simulink model "35 Bus Network Electricity Transmission Model"  (R2023b)
settings: Solver=VariableStepAuto  StartTime=0.0  StopTime=1  RelTol=1e-3
model workspace (MAT data in the model file):
  T_set = 0.0001
  Tp = 5e-05
undefined symbols (not defined in the file): D1, D11, Delta, DiscIntNeverNeededParam
libraries: spsSeriesRLCBranchLib x57, spsLoadFlowBusLib x35, spsThreePhaseSeriesRLCLoadLib x28, spsThreePhaseTransformerTwoWindingsLib x22, spsDistributedParametersLineLib x22, spsGenericPowerSystemStabilizerLib x20, spsThreePhaseVIMeasurementLib x14, spsSynchronousMachinepuStandardLib x10, spsExcitationSystemLib x10, spsHydraulicTurbineandGovernorLib x10, spsFourierLib x8, spsMeanLib x8
(part 1 of 8)
settings Model: Creator=3.22  LastModifiedBy=3.22

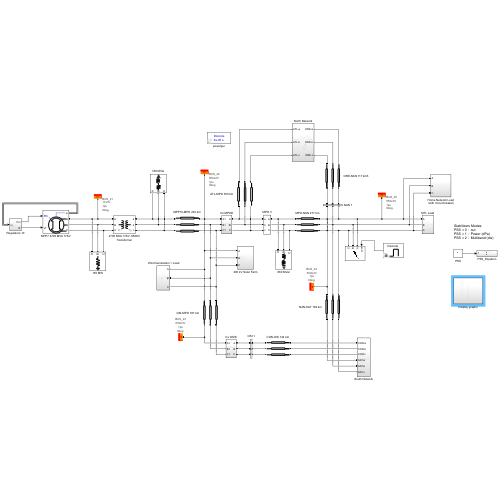
[thumbnail: Simulink's stored preview of the top-level diagram]
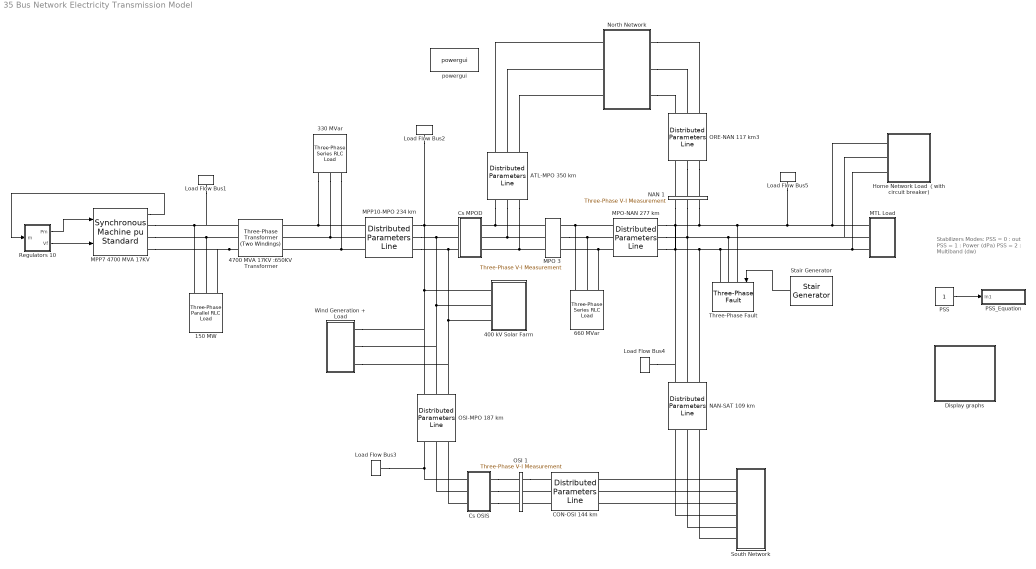
== system 35 Bus Network Electricity Transmission Model ==
  note: Stabilizers Modes:
      | PSS = 0 :  out
      | PSS = 1 :  Power (dPa)
      | PSS = 2 :  Multiband (dw)
  " Wind Generation + Load" : Subsystem
  150 MW : spsThreePhaseParallelRLCLoadLib/Three-Phase Parallel RLC Load  LConnTagsString=A|B|C  Configuration=Y (grounded)  NominalVoltage=17000  Vabc=[1e3 1e3 1e3]  Vabcp=[1e3 1e3 1e3]  NominalFrequency=60  UnbalancedPower=off  ActivePower=150e6  InductivePower=0  CapacitivePower=0  Pabc=[10e3 9e3 11e3]  QLabc=[100 90 110]  QCabc=[100 90 110]  Pabcp=[10e3 9e3 11e3]  QLabcp=[100 90 110]  QCabcp=[100 90 110]  Measurements=None  LoadType=constant Z
  330 MVar : spsThreePhaseSeriesRLCLoadLib/Three-Phase Series RLC Load  LConnTagsString=A|B|C  Configuration=Y (grounded)  NominalVoltage=650e3  Vabc=[1e3 1e3 1e3]  Vabcp=[1e3 1e3 1e3]  NominalFrequency=60  UnbalancedPower=off  ActivePower=1100e3  InductivePower=330e6  CapacitivePower=0  Pabc=[10e3 9e3 11e3]  QLabc=[100 90 110]  QCabc=[100 90 110]  Pabcp=[10e3 9e3 11e3]  QLabcp=[100 90 110]  QCabcp=[100 90 110]  Measurements=None  LoadType=constant Z
  400 kV Solar Farm : Subsystem
  "4700 MVA 17KV :650KV Transformer " : spsThreePhaseTransformerTwoWindingsLib/Three-Phase Transformer (Two Windings)  Winding1Connection=Delta (D1)  Winding2Connection=Yg  CoreType=Three single-phase transformers  SetSaturation=off  Hysteresis=off  DataFile='hysteresis'  SetInitialFlux=off  Measurements=None  UNITS=pu  NominalPower=[ 4700e6 , 60 ]  Winding1=[ 17e3 , 0.002 , 0.08 ]  Winding2=[ 650e3 , 0.002 , 0.08 ]  Rm=500  Lm=500  L0=0.5  Saturation=[ 0,0 ; 0.0024,1.2 ; 1.0,1.52 ]  InitialFluxes=[ 0.8 , -0.8 , 0.7 ]  BreakLoop=off  DiscreteSolver=Trapezoidal iterative  DataType=off  TransfoNumber=1
  660 MVar : spsThreePhaseSeriesRLCLoadLib/Three-Phase Series RLC Load  LConnTagsString=A|B|C  Configuration=Y (grounded)  NominalVoltage=650e3  Vabc=[1e3 1e3 1e3]  Vabcp=[1e3 1e3 1e3]  NominalFrequency=60  UnbalancedPower=off  ActivePower=2200e3  InductivePower=660e6  CapacitivePower=0  Pabc=[10e3 9e3 11e3]  QLabc=[100 90 110]  QCabc=[100 90 110]  Pabcp=[10e3 9e3 11e3]  QLabcp=[100 90 110]  QCabcp=[100 90 110]  Measurements=None  LoadType=constant Z
  ATL-MPO 350 km : spsDistributedParametersLineLib/Distributed Parameters Line  Phases=3  Length=350  Frequency=60  Resistance=[0.01273 0.3864]/6  Inductance="[0.9337e-3  4.1264e-3]/6"  Capacitance=[12.74e-9 7.751e-9]*6  x1=[-0.00198 -4.66537973862611e-08 -283995.035900817 -140929.158887352;-0.00192 -4.56218918231529e-08 -280734.893310355 -147316.404665037;-0.00186 -4.45666452571923e-08 -277331.121561091 -153628.280648;-0.0018 -4.34885975720212e-08 -273785.462085546 -159861.557563859;-0.00174 -4.23883003167554e-08 -270099.728908624 -166013.046352967;-0.00168 -4.12663164238018e-08 -266275.807719524 -172079.599799993;-0.00162 -4.0123219920852e-08 -262315.654906983 -178058.114144095;-0.00156 -3.89595956371987e-08 -258221.296558356 -183945.530666865;-0.0015 -3.77760389045269e-08 -253994.827423029 -189738.837257224;-0.00144 -3.65731552523307e-08 -249638.409840707 -195435.069952471;-0.00138 -3.53515600981131e-08 -245154.272635124 -201031.314454706;-0.00132 -3.41118784325276e-08 -240544.70997373 -206524.707621834;-0.00126 -3.2854744499621e-08 -235812.080193958 -211912.438932405;-0.0012 -3.15808014723424e-08 -230958.804596653 -217191.751923527;-0.00114 -3.02907011234846e-08 -225987.366207288 -222359.945601122;-0.00108 -2.89851034922241e-08 -220900.308505605 -227414.375821808;-0.00102 -2.76646765464339e-08 -215700.234124322 -232352.45664569;-0.00096 -2.63300958409381e-08 -210389.803517579 -237171.661659371;-0.0009 -2.49820441718858e-08 -204971.7335998 -241869.52526852;-0.00084 -2.36212112274201e-08 -199448.796355669 -246443.643959306;-0.00078 -2.22482932348207e-08 -193823.817421933 -250891.677528087;-0.00072 -2.08639926043011e-08 -188099.674641751 -255211.3502787;-0.00066 -1.94690175696429e-08 -182279.29659234 -259400.452186747;-0.0006 -1.806408182585e-08 -176365.661086658 -263456.840030286;-0.00054 -1.66499041640091e-08 -170361.793649902 -267378.438486342;-0.00048 -1.52272081035431e-08 -164270.76597159 -271163.241192684;-0.00042 -1.37967215220448e-08 -158095.694334033 -274809.31177431;-0.00036 -1.23591762828818e-08 -151839.738017982 -278314.784834141;-0.0003 -1.09153078607611e-08 -145506.097686284 -281677.866907385;-0.00024 -9.46585496544719e-09 -139098.013746368 -284896.83737911;-0.00018 -8.01155916382403e-09 -132618.764692382 -287970.049364544;-0.00012 -6.55316450049607e-09 -126071.665427867 -290895.930551648;-6e-05 -5.0914171171211e-09 -119460.065569783 -293672.984005544]  x2=[-0.00198 -4.73470407763487e-08 -244678.153400783 -153858.077281588;-0.00192 -4.70683207225062e-08 -241135.650149882 -159352.765994398;-0.00186 -4.67655196460595e-08 -237469.77744469 -164765.926887624;-0.0018 -4.64387924656344e-08 -233682.41081342 -170094.790488131;-0.00174 -4.60883063408937e-08 -229775.487942824 -175336.630450834;-0.00168 -4.5714240587015e-08 -225751.007686833 -180488.764953549;-0.00162 -4.53167865829499e-08 -221611.02904391 -185548.558069066;-0.00156 -4.48961476735111e-08 -217357.670103628 -190513.421113731;-0.0015 -4.44525390653371e-08 -212993.106963013 -195380.813971871;-0.00144 -4.39861877167887e-08 -208519.572613215 -200148.24639536;-0.00138 -4.34973322218332e-08 -203939.35579707 -204813.27927768;-0.00132 -4.29862226879746e-08 -199254.799838133 -209373.525901807;-0.00126 -4.24531206082949e-08 -194468.301441793 -213826.653161304;-0.0012 -4.18982987276684e-08 -189582.309469075 -218170.382753982;-0.00114 -4.13220409032214e-08 -184599.323683754 -222402.492347517;-0.00108 -4.07246419591047e-08 -179521.893473433 -226520.816716443;-0.00102 -4.01064075356569e-08 -174352.616545228 -230523.248849912;-0.00096 -3.94676539330326e-08 -169094.137596732 -234407.74102969;-0.0009 -3.88087079493778e-08 -163749.146962942 -238172.305877801;-0.00084 -3.81299067136336e-08 -158320.379239828 -241815.017373306;-0.00078 -3.74315975130551e-08 -152810.611885272 -245334.011837695;-0.00072 -3.67141376155325e-08 -147222.66379806 -248727.488888376;-0.00066 -3.59778940868065e-08 -141559.393875686 -251993.712359787;-0.0006 -3.52232436026707e-08 -135823.699551689 -255131.011191646;-0.00054 -3.4450572256257e-08 -130018.515313268 -258137.7802839;-0.00048 -3.36602753605036e-08 -124146.811199946 -261012.481317923;-0.00042 -3.28527572459055e-08 -118211.591284045 -263753.643543548;-0.00036 -3.20284310536511e-08 -112215.892133745 -266359.864531529;-0.0003 -3.11877185242524e-08 -106162.781259517 -268829.810891052;-0.00024 -3.03310497817739e-08 -100055.355544735 -271162.218951918;-0.00018 -2.94588631137736e-08 -93896.739661245 -273355.895411067;-0.00012 -2.85716047470672e-08 -87690.0844707324 -275409.717943088;-6e-05 -2.76697286194296e-08 -81438.5654126781 -277322.635774423]  x3=[-0.00198 -1.15739742869573e-10 -7510.86676188477 -3625.13536494991;-0.00192 -1.13432270648557e-10 -7426.95305478795 -3794.08593924927;-0.00186 -1.11066764381889e-10 -7339.23958127399 -3961.09538907547;-0.0018 -1.08644434306286e-10 -7247.7712171767 -4126.07826930798;-0.00174 -1.06166519730574e-10 -7152.59475940128 -4288.95017165676;-0.00168 -1.03634288401635e-10 -7053.7589019822 -4449.62776784703;-0.00162 -1.01049035855809e-10 -6951.31421117039 -4608.02885225161;-0.00156 -9.84120847560678e-11 -6845.31309956262 -4764.07238394879;-0.0015 -9.57247842153189e-11 -6735.80979928628 -4917.6785281844;-0.00144 -9.29885091061748e-11 -6622.86033425316 -5068.76869721674;-0.00138 -9.02046593575419e-11 -6506.52249149665 -5217.26559052351;-0.00132 -8.73746592383912e-11 -6386.85579160679 -5363.09323435019;-0.00126 -8.4499956629076e-11 -6263.9214582784 -5506.1770205796;-0.0012 -8.15820222805698e-11 -6137.78238698801 -5646.44374490283;-0.00114 -7.86223490620024e-11 -6008.50311281525 -5783.82164427189;-0.00108 -7.56224511968808e-11 -5876.1497774256 -5918.240433615;-0.00102 -7.25838634883847e-11 -5740.79009523106 -6049.63134179576;-0.00096 -6.95081405341324e-11 -5602.49331874619 -6177.92714679772;-0.0009 -6.63968559308201e-11 -5461.33020315728 -6303.06221011642;-0.00084 -6.32516014691407e-11 -5317.37297012266 -6424.97251034122;-0.00078 -6.00739863193944e-11 -5170.69527082276 -6543.59567590988;-0.00072 -5.68656362082076e-11 -5021.37214827885 -6658.87101701901;-0.00066 -5.36281925867804e-11 -4869.47999895959 -6770.73955667404;-0.0006 -5.03633117910908e-11 -4715.09653369522 -6879.14406086299;-0.00054 -4.70726641944819e-11 -4558.30073791924 -6984.02906783844;-0.00048 -4.37579333530683e-11 -4399.17283125803 -7085.34091649276;-0.00042 -4.04208151443976e-11 -4237.79422648898 -7183.02777381216;-0.00036 -3.70630168998082e-11 -4074.24748788822 -7277.03966139538;-0.0003 -3.3686256530927e-11 -3908.61628898922 -7367.3284810236;-0.00024 -3.02922616507542e-11 -3740.98536977385 -7453.84803926836;-0.00018 -2.68827686897843e-11 -3571.44049331784 -7536.55407112494;-0.00012 -2.34595220076162e-11 -3400.06840191282 -7615.40426265923;-6e-05 -2.00242730005068e-11 -3226.95677268734 -7690.35827265625]  x4=[-0.00198 -7.16737734589059e-10 -5560.43523467954 -135.899816413835;-0.00192 -7.1591261080325e-10 -5555.93855175485 -261.62884284291;-0.00186 -7.1472121289721e-10 -5548.59934800515 -387.224015121641;-0.0018 -7.13164150412122e-10 -5538.42137830268 -512.621076439158;-0.00174 -7.11242219969926e-10 -5525.40984988481 -637.755871341821;-0.00168 -7.08956404865747e-10 -5509.5714196899 -762.564378556332;-0.00162 -7.06307874564831e-10 -5490.91419095151 -886.982743744204;-0.00156 -7.03297984104218e-10 -5469.44770905259 -1010.94731217082;-0.0015 -6.99928273399485e-10 -5445.18295664195 -1134.39466127237;-0.00144 -6.96200466456894e-10 -5418.13234801529 -1257.26163310401;-0.00138 -6.92116470491358e-10 -5388.3097227638 -1379.48536665263;-0.00132 -6.87678374950676e-10 -5355.73033869363 -1501.00332999771;-0.00126 -6.82888450446534e-10 -5320.41086401966 -1621.75335230382;-0.0012 -6.77749147592816e-10 -5282.36936883778 -1741.67365562832;-0.00114 -6.72263095751826e-10 -5241.62531587983 -1860.70288652818;-0.00108 -6.66433101689054e-10 -5198.19955055618 -1978.78014744946;-0.00102 -6.60262148137191e-10 -5152.11429029078 -2095.84502788364;-0.00096 -6.53753392270099e-10 -5103.39311315434 -2211.8376352748;-0.0009 -6.46910164087548e-10 -5052.06094580135 -2326.69862566169;-0.00084 -6.39735964711525e-10 -4998.14405071713 -2440.36923403925;-0.00078 -6.32234464594993e-10 -4941.67001278149 -2552.79130442383;-0.00072 -6.24409501644025e-10 -4882.66772515574 -2663.90731960691;-0.00066 -6.16265079254255e-10 -4821.16737450048 -2773.66043058193;-0.0006 -6.07805364262669e-10 -4757.20042553149 -2881.99448562931;-0.00054 -5.99034684815774e-10 -4690.79960492184 -2988.85405904471;-0.00048 -5.89957528155239e-10 -4621.9988845583 -3094.18447949583;-0.00042 -5.80578538322139e-10 -4550.83346416071 -3197.93185799329;-0.00036 -5.70902513780975e-10 -4477.33975327311 -3300.0431154612;-0.0003 -5.60934404964694e-10 -4401.55535263602 -3400.46600989346;-0.00024 -5.50679311741958e-10 -4323.51903494912 -3499.14916308168;-0.00018 -5.40142480807951e-10 -4243.2707250345 -3596.04208690122;-0.00012 -5.29329303000077e-10 -4160.85147941032 -3691.09520914188;-6e-05 -5.18245310539908e-10 -4076.30346528558 -3784.25989886994]  x5=0.0019793954844851  V1=[4.219e-16 0.0001256 0.0001256;377 377 377;2.896 1.02 -0.5506]  V2=[3.447e-16 8.016e-05 8.016e-05;377 377 377;2.788 1.015 -0.5555]  I1=[4.128e-19 5.188e-07 5.188e-07;377 377 377;2.697 1.572 0.0007381]  I2=[5.884e-19 5.436e-07 5.436e-07;377 377 377;2.289 0.05248 -1.518]  nHarmo=1  Measurements=None  Decoupling=off  VsMag0=0  VrMag0=0  VsAngle0=0  VrAngle0=0  IsMag0=0  IrMag0=0  IsAngle0=0  IrAngle0=0
      settings: LibrarySourceBlock=sps_lib/Power Grid Elements/Distributed Parameters Line
  CON-OSI 144 km : spsDistributedParametersLineLib/Distributed Parameters Line  Phases=3  Length=144  Frequency=60  Resistance=[0.01273 0.3864]/6  Inductance="[0.9337e-3  4.1264e-3]/6"  Capacitance=[12.74e-9 7.751e-9]*6  x1=[-0.00084 1.58878300947761e-08 0 0;-0.00078 1.81135659339013e-08 0 0;-0.00072 2.03300345379945e-08 0 0;-0.00066 2.25361019207623e-08 0 0;-0.0006 2.4730639417368e-08 0 0;-0.00054 2.69125242618782e-08 -153418.27699203 -260460.282018713;-0.00048 2.90806401616898e-08 -147488.056603015 -263863.63509505;-0.00042 3.12338778686461e-08 -141482.378598976 -267131.990660033;-0.00036 3.33711357465492e-08 -135404.315595752 -270263.676562563;-0.0003 3.54913203347766e-08 -129256.977242685 -273257.090574265;-0.00024 3.75933469077166e-08 -123043.508631666 -276110.701209219;-0.00018 3.96761400297334e-08 -116767.088688049 -278823.048507495;-0.00012 4.17386341053802e-08 -110430.928544252 -281392.744782097;-6e-05 4.37797739245774e-08 -104038.269896882 -283818.475328928]  x2=[-0.00084 2.59938982630843e-08 0 0;-0.00078 2.7994091738396e-08 0 0;-0.00072 2.9979962919103e-08 0 0;-0.00066 3.19504957968145e-08 0 0;-0.0006 3.39046822104992e-08 0 0;-0.00054 3.58415223622784e-08 -143552.051614192 -254203.94929145;-0.00048 3.77600253289419e-08 -137765.858511586 -257385.752758705;-0.00042 3.9659209568922e-08 -131909.181850144 -260435.872918908;-0.00036 4.15381034244688e-08 -125985.018013867 -263352.749274224;-0.0003 4.33957456187677e-08 -119996.397914438 -266134.889496811;-0.00024 4.52311857477469e-08 -113946.385440558 -268780.870192325;-0.00018 4.70434847663213e-08 -107838.075890399 -271289.337628149;-0.00012 4.88317154688256e-08 -101674.594387996 -273659.008425992;-6e-05 5.05949629633897e-08 -95459.0942843738 -275888.670218487]  x3=[-0.00084 3.07553029750544e-10 0 0;-0.00078 3.29548959067833e-10 0 0;-0.00072 3.51376285048298e-10 0 0;-0.00066 3.73023840428645e-10 0 0;-0.0006 3.94480549919541e-10 0 0;-0.00054 4.15735435871936e-10 -3139.71318404474 -6567.77181842436;-0.00048 4.3677762389343e-10 -2990.36305476603 -6637.10518863291;-0.00042 4.57596348411819e-10 -2839.48300049295 -6703.04289318734;-0.00036 4.78180958182951e-10 -2687.1502142492 -6765.55119713963;-0.0003 4.98520921740109e-10 -2533.44263230302 -6824.59812008645;-0.00024 5.18605832782097e-10 -2378.43889429351 -6880.15345253095;-0.00018 5.384254154973e-10 -2222.21830299718 -6932.18877133853;-0.00012 5.57969529820977e-10 -2064.86078375517 -6980.67745427856;-6e-05 5.77228176623106e-10 -1906.44684358194 -7025.5946936449]  x4=[-0.00084 -2.09296979855395e-10 0 0;-0.00078 -1.97214230323626e-10 0 0;-0.00072 -1.85030582347523e-10 0 0;-0.00066 -1.72752269306518e-10 0 0;-0.0006 -1.60385573012442e-10 0 0;-0.00054 -1.47936820495628e-10 -4476.02404663198 -4165.00505473071;-0.00048 -1.3541238076789e-10 -4380.67668178872 -4265.17699903546;-0.00042 -1.22818661564018e-10 -4283.08808180945 -4363.1667999761;-0.00036 -1.10162106063462e-10 -4183.30817482517 -4458.92432415982;-0.0003 -9.74491895938823e-11 -4081.38801008 -4552.40058026784;-0.00024 -8.46864163182524e-11 -3977.37973181349 -4643.54774412032;-0.00018 -7.1880315907209e-11 -3871.33655258266 -4732.319183144;-0.00012 -5.9037440198352e-11 -3763.31272603746 -4818.66948023038;-6e-05 -4.6164359844203e-11 -3653.36351916359 -4902.55445697191]  x5=0.000814379856473869  V1=[3.066e-13 0.3294 0.3294;377 377 377;-0.5534 -1.851 2.861]  V2=[2.167e-13 0.2213 0.2213;377 377 377;-0.5727 -1.852 2.86]  I1=[4.19e-16 0.002316 0.002316;377 377 377;0.2564 -0.79 -2.361]  I2=[5.677e-16 0.002387 0.002387;377 377 377;-1.374 -3.038 1.674]  nHarmo=1  Measurements=None  Decoupling=off  VsMag0=0  VrMag0=0  VsAngle0=0  VrAngle0=0  IsMag0=0  IrMag0=0  IsAngle0=0  IrAngle0=0
      settings: LibrarySourceBlock=sps_lib/Power Grid Elements/Distributed Parameters Line
  Cs MPOD : Subsystem
  Cs OSIS : Subsystem
  Display graphs : Subsystem
  Home Network Load （with circuit breaker) : Subsystem
  Load Flow Bus1 : spsLoadFlowBusLib/Load Flow Bus  LConnTagsString=a  Phases=single  Connectors=on one side  ID=BUS_21  Vbase=17e3  Vref=1  Vangle=0  VLF=1  VLFb=1  VLFc=1  angleLF=0  angleLFb=0  angleLFc=0
  Load Flow Bus2 : spsLoadFlowBusLib/Load Flow Bus  LConnTagsString=a  Phases=single  Connectors=on one side  ID=BUS_22  Vbase=650e3  Vref=1  Vangle=0  VLF=1  VLFb=1  VLFc=1  angleLF=0  angleLFb=0  angleLFc=0
  Load Flow Bus3 : spsLoadFlowBusLib/Load Flow Bus  LConnTagsString=a  Phases=single  Connectors=on one side  ID=BUS_23  Vbase=650e3  Vref=1  Vangle=0  VLF=1  VLFb=1  VLFc=1  angleLF=0  angleLFb=0  angleLFc=0
  Load Flow Bus4 : spsLoadFlowBusLib/Load Flow Bus  LConnTagsString=a  Phases=single  Connectors=on one side  ID=BUS_24  Vbase=650e3  Vref=1  Vangle=0  VLF=1  VLFb=1  VLFc=1  angleLF=0  angleLFb=0  angleLFc=0
  Load Flow Bus5 : spsLoadFlowBusLib/Load Flow Bus  LConnTagsString=a  Phases=single  Connectors=on one side  ID=BUS_25  Vbase=650e3  Vref=1  Vangle=0  VLF=1  VLFb=1  VLFc=1  angleLF=0  angleLFb=0  angleLFc=0
  MPO 3 : spsThreePhaseVIMeasurementLib/Three-Phase V-I Measurement  VoltageMeasurement=no  SetLabelV=off  LabelV=Vabc_MPO3  Vpu=off  VpuLL=off  CurrentMeasurement=no  SetLabelI=off  LabelI=Iabc  Ipu=off  Pbase=100e6  Vbase=500e3  OutputType=Complex  PhasorSimulation=off  PSBequivalent=0
  MPO-NAN 277 km : spsDistributedParametersLineLib/Distributed Parameters Line  Phases=3  Length=277  Frequency=60  Resistance=[0.01273 0.3864]/6  Inductance="[0.9337e-3  4.1264e-3]/6"  Capacitance=[12.74e-9 7.751e-9]*6  x1=[-0.00162 -4.0123219920852e-08 -262315.654906984 -178058.114144095;-0.00156 -3.89595956371987e-08 -258221.296558356 -183945.530666865;-0.0015 -3.77760389045269e-08 -253994.827423029 -189738.837257224;-0.00144 -3.65731552523307e-08 -249638.409840707 -195435.069952471;-0.00138 -3.53515600981131e-08 -245154.272635124 -201031.314454706;-0.00132 -3.41118784325276e-08 -240544.70997373 -206524.707621834;-0.00126 -3.2854744499621e-08 -235812.080193958 -211912.438932405;-0.0012 -3.15808014723424e-08 -230958.804596653 -217191.751923527;-0.00114 -3.02907011234846e-08 -225987.366207288 -222359.945601122;-0.00108 -2.89851034922241e-08 -220900.308505605 -227414.375821808;-0.00102 -2.76646765464339e-08 -215700.234124322 -232352.45664569;-0.00096 -2.63300958409381e-08 -210389.803517579 -237171.661659371;-0.0009 -2.49820441718858e-08 -204971.7335998 -241869.52526852;-0.00084 -2.36212112274201e-08 -199448.796355669 -246443.643959306;-0.00078 -2.22482932348207e-08 -193823.817421933 -250891.677528087;-0.00072 -2.08639926043011e-08 -188099.674641751 -255211.3502787;-0.00066 -1.94690175696429e-08 -182279.29659234 -259400.452186747;-0.0006 -1.806408182585e-08 -176365.661086658 -263456.840030286;-0.00054 -1.66499041640091e-08 -170361.793649902 -267378.438486342;-0.00048 -1.52272081035431e-08 -164270.76597159 -271163.241192684;-0.00042 -1.37967215220448e-08 -158095.694334033 -274809.31177431;-0.00036 -1.23591762828818e-08 -151839.738017982 -278314.784834141;-0.0003 -1.09153078607611e-08 -145506.097686284 -281677.866907385;-0.00024 -9.46585496544719e-09 -139098.013746368 -284896.83737911;-0.00018 -8.01155916382403e-09 -132618.764692382 -287970.049364544;-0.00012 -6.55316450049607e-09 -126071.665427867 -290895.930551648;-6e-05 -5.0914171171211e-09 -119460.065569783 -293672.984005544]  x2=[-0.00162 1.18325766507148e-08 -199728.896429736 -137284.436590295;-0.00156 1.16737896771227e-08 -196572.752502674 -141766.721761987;-0.0015 1.15090301770249e-08 -193316.038323184 -146176.476459277;-0.00144 1.13383824444261e-08 -189960.420086419 -150511.44457018;-0.00138 1.11619337858596e-08 -186507.614588672 -154769.408244909;-0.00132 1.09797744757194e-08 -182959.388349038 -158948.189030571;-0.00126 1.07919977100745e-08 -179317.556705623 -163045.648985699;-0.0012 1.05986995589879e-08 -175583.98288679 -167059.691774069;-0.00114 1.03999789173655e-08 -171760.577057894 -170988.26373722;-0.00108 1.01959374543595e-08 -167849.295344004 -174829.354945142;-0.00102 9.98667956135251e-09 -163852.138829117 -178581.0002246;-0.00096 9.77231229854936e-09 -159771.152532367 -182241.280164545;-0.0009 9.5529453402027e-09 -155608.424361749 -185808.322098126;-0.00084 9.32869091850185e-09 -151366.084045914 -189280.301060779;-0.00078 9.09966376615271e-09 -147046.302044559 -192655.440723912;-0.00072 8.86598105767836e-09 -142651.288437973 -195932.014303706;-0.00066 8.6277623494704e-09 -138183.291796331 -199108.345444576;-0.0006 8.38512951862173e-09 -133644.598029271 -202182.809076817;-0.00054 8.13820670057196e-09 -129037.529216392 -205153.832248025;-0.00048 7.8871202255974e-09 -124364.442419226 -208019.894927849;-0.00042 7.63199855417821e-09 -119627.728475328 -210779.530785662;-0.00036 7.37297221127558e-09 -114829.810775075 -213431.327940766;-0.0003 7.11017371955279e-09 -109973.144021819 -215973.929684739;-0.00024 6.84373753157418e-09 -105060.212976012 -218406.035175546;-0.00018 6.57379996101669e-09 -100093.531183956 -220726.400103077;-0.00012 6.30049911292928e-09 -95075.6396918308 -222933.837325761;-6e-05 6.02397481307586e-09 -90009.1057456434 -225027.217477925]  x3=[-0.00162 4.93435604063458e-10 -3788.75201737561 -6671.92895558431;-0.00156 5.11032265207607e-10 -3636.87987138775 -6755.91530093014;-0.0015 5.28367472802086e-10 -3483.14703045588 -6836.44519517306;-0.00144 5.45432357834371e-10 -3327.63214714207 -6913.47743773114;-0.00138 5.62218189593956e-10 -3170.4147857342 -6986.9726174857;-0.00132 5.78716380139148e-10 -3011.57538153943 -7056.89313294475;-0.00126 5.94918488690811e-10 -2851.19519973195 -7123.20321148059;-0.0012 6.1081622595083e-10 -2689.35629377625 -7185.86892763178;-0.00114 6.26401458343066e-10 -2526.14146344707 -7244.85822045999;-0.00108 6.41666212174646e-10 -2361.63421246746 -7300.14090995304;-0.00102 6.5660267771545e-10 -2195.91870578677 -7351.68871246545;-0.00096 6.71203213193711e-10 -2029.07972652029 -7399.47525518898;-0.0009 6.85460348705693e-10 -1861.20263257263 -7443.47608964538;-0.00084 6.99366790037426e-10 -1692.37331296708 -7483.66870419468;-0.00078 7.12915422396564e-10 -1522.67814390316 -7520.03253555263;-0.00072 7.26099314052442e-10 -1352.20394456495 -7552.54897931115;-0.00066 7.38911719882477e-10 -1181.03793270285 -7581.20139945681;-0.0006 7.51346084823102e-10 -1009.26768001131 -7605.975136882;-0.00054 7.63396047223451e-10 -836.981067325554 -7626.85751688491;-0.00048 7.75055442100105e-10 -664.26623966012 -7643.83785565405;-0.00042 7.86318304291202e-10 -491.211561112247 -7656.90746573436;-0.00036 7.97178871508331e-10 -317.905569653163 -7666.05966047182;-0.0003 8.07631587284626e-10 -144.436931830425 -7671.28975743448;-0.00024 8.17671103817549e-10 29.105602595525 -7672.5950808081;-0.00018 8.27292284704935e-10 202.633246057378 -7669.97496276512;-0.00012 8.36490207572862e-10 376.057218606315 -7663.43074380636;-6e-05 8.45260166594032e-10 549.288793333476 -7652.96577207514]  x4=[-0.00162 -8.02734838898159e-10 -7615.15319529617 1603.79602779119;-0.00156 -8.14433614742137e-10 -7649.47842680911 1431.14943236951;-0.0015 -8.2571571129981e-10 -7679.89004381277 1257.77063445362;-0.00144 -8.3657535644211e-10 -7706.37248716197 1083.74833784022;-0.00138 -8.47006994173919e-10 -7728.91220794935 909.171575551815;-0.00132 -8.57005287476619e-10 -7747.49767443726 734.129664285796;-0.00126 -8.66565121038609e-10 -7762.11937795764 558.712158718372;-0.0012 -8.75681603872393e-10 -7772.76983777677 383.008805686735;-0.00114 -8.84350071816901e-10 -7779.44360492263 207.109498272919;-0.00108 -8.92566089923756e-10 -7782.13726497261 31.1042298128429;-0.00102 -9.00325454726282e-10 -7780.84943980048 -144.916952145947;-0.00096 -9.07624196390067e-10 -7775.58078828137 -320.863991914259;-0.0009 -9.14458580744013e-10 -7766.33400595477 -496.646871735425;-0.00084 -9.20825111190799e-10 -7753.11382364536 -672.175657840031;-0.00078 -9.26720530495807e-10 -7735.92700504271 -847.360546457708;-0.00072 -9.32141822453587e-10 -7714.78234324079 -1022.11190976239;-0.00066 -9.37086213431e-10 -7689.69065623927 -1196.34034172759;-0.0006 -9.41551173786259e-10 -7660.66478140888 -1369.95670386813;-0.00054 -9.45534419163143e-10 -7627.7195689235 -1542.87217084508;-0.00048 -9.49033911659716e-10 -7590.87187416262 -1714.99827591043;-0.00042 -9.52047860870954e-10 -7550.14054908772 -1886.2469561683;-0.00036 -9.54574724804748e-10 -7505.54643259736 -2056.53059762955;-0.0003 -9.5661321067082e-10 -7457.11233986553 -2225.76208003674;-0.00024 -9.58162275542132e-10 -7404.86305066903 -2393.85482143643;-0.00018 -9.59221126888474e-10 -7348.82529670967 -2560.72282247613;-0.00012 -9.59789222981931e-10 -7289.02774793783 -2726.28071040312;-6e-05 -9.59866273174045e-10 -7225.5009978844 -2890.4437827428]  x5=0.00156655014057821  V1=[4.219e-16 0.0001256 0.0001256;377 377 377;3.052 1.115 -0.4557]  V2=[4.095e-15 0.006804 0.006804;377 377 377;-1.109 1.061 -0.5096]  I1=[9.849e-18 6.958e-05 6.958e-05;377 377 377;-2.423 -0.4689 -2.04]  I2=[7.867e-18 6.871e-05 6.871e-05;377 377 377;0.191 2.298 0.7273]  nHarmo=1  Measurements=None  Decoupling=off  VsMag0=0  VrMag0=0  VsAngle0=0  VrAngle0=0  IsMag0=0  IrMag0=0  IsAngle0=0  IrAngle0=0
      settings: LibrarySourceBlock=sps_lib/Power Grid Elements/Distributed Parameters Line
  MPP10-MPO 234 km : spsDistributedParametersLineLib/Distributed Parameters Line  Phases=3  Length=234  Frequency=60  Resistance=[0.01273 0.3864]/6  Inductance="[0.9337e-3  4.1264e-3]/6"  Capacitance=[12.74e-9 7.751e-9]*6  x1=[-0.00138 4.11714216300909e-08 -184319.317778621 -182101.613478184;-0.00132 4.15737418012643e-08 -180153.464177139 -186223.909700941;-0.00126 4.19547920779379e-08 -175895.440734531 -190250.930330474;-0.0012 4.23143775077489e-08 -171547.425934268 -194180.615068617;-0.00114 4.26523141201471e-08 -167111.644301066 -198010.953416045;-0.00108 4.29684290205174e-08 -162590.365262771 -201739.985700884;-0.00102 4.32625604786354e-08 -157985.901989283 -205365.804081312;-0.00096 4.35345580114124e-08 -153300.610209094 -208886.553521648;-0.0009 4.37842824598846e-08 -148536.887004052 -212300.432741423;-0.00084 4.40116060604098e-08 -143697.169582973 -215605.695136946;-0.00078 4.42164125100335e-08 -138783.934034716 -218800.649674902;-0.00072 4.43985970259918e-08 -133799.694061375 -221883.661757514;-0.00066 4.45580663993198e-08 -128746.999692219 -224853.154058831;-0.0006 4.46947390425395e-08 -123628.435979048 -227707.607331724;-0.00054 4.48085450314012e-08 -118446.621673641 -230445.561185152;-0.00048 4.48994261406581e-08 -113204.207887942 -233065.614831334;-0.00042 4.49673358738555e-08 -107903.876737716 -235566.427802411;-0.00036 4.50122394871189e-08 -102548.339970315 -237946.720636257;-0.0003 4.50341140069302e-08 -97140.3375773108 -240205.275531076;-0.00024 4.50329482418808e-08 -91682.6363926547 -242340.93696845;-0.00018 4.50087427883977e-08 -86178.0286771197 -244352.612304525;-0.00012 4.4961510030438e-08 -80629.3306897267 -246239.272329028;-6e-05 4.48912741331536e-08 -75039.381246894 -247999.951791828]  x2=[-0.00138 -1.43218533750548e-08 -224905.507139955 -193613.771522024;-0.00132 -1.21580910624106e-08 -220468.891984961 -198651.085236779;-0.00126 -9.98810844572322e-09 -215919.48087103 -203586.765385676;-0.0012 -7.81301572819595e-09 -211259.601360953 -208418.286783552;-0.00114 -5.63392572745422e-09 -206491.637535191 -213143.177534782;-0.00108 -3.45195330620732e-09 -201618.028772139 -217759.020297952;-0.00102 -1.26821480186421e-09 -196641.268500095 -222263.453522613;-0.00096 9.16172544605437e-10 -191563.902921573 -226654.172657496;-0.0009 3.10009116027235e-09 -186388.529710622 -230928.93132956;-0.00084 5.28242371201857e-09 -181117.796683807 -235085.54249328;-0.00078 7.46205367818575e-09 -175754.400445537 -239121.879549578;-0.00072 9.63786591980827e-09 -170301.085008431 -243035.877433835;-0.00066 1.18087472511389e-08 -164760.640389433 -246825.53367241;-0.0006 1.39735870091754e-08 -159135.901182384 -250488.909407147;-0.00054 1.61312776218957e-08 -153429.745107798 -254024.130387328;-0.00048 1.82807151749129e-08 -147645.091540558 -257429.387928577;-0.00042 2.04207999762579e-08 -141784.900016319 -260702.939838213;-0.00036 2.2550437119002e-08 -135852.168717347 -263843.111306591;-0.0003 2.46685370414318e-08 -129849.932938601 -266848.295763965;-0.00024 2.67740160844891e-08 -123781.263534812 -269716.955702437;-0.00018 2.88657970461907e-08 -117649.265349384 -272447.623462575;-0.00012 3.09428097327448e-08 -111457.075625894 -275038.901984296;-6e-05 3.30039915060823e-08 -105207.862403025 -277489.465521627]  x3=[-0.00138 -1.10520599308306e-09 -5618.33788115026 -427.368141304456;-0.00132 -1.11289338916343e-09 -5607.23405337276 -554.332230159398;-0.00126 -1.120011408422e-09 -5593.26146104379 -681.012712402508;-0.0012 -1.1265564091486e-09 -5576.42725279976 -807.344775958284;-0.00114 -1.1325250427999e-09 -5556.74004133267 -933.263787008664;-0.00108 -1.13791425571265e-09 -5534.20989898369 -1058.70532306088;-0.00102 -1.14272129066594e-09 -5508.84835258994 -1183.60520590719;-0.00096 -1.14694368829186e-09 -5480.66837758719 -1307.89953445965;-0.0009 -1.15057928833377e-09 -5449.68439137136 -1431.52471744308;-0.00084 -1.15362623075151e-09 -5415.91224592232 -1554.41750592952;-0.00078 -1.15608295667303e-09 -5379.36921969371 -1676.5150256976;-0.00072 -1.15794820919196e-09 -5340.07400877299 -1797.7548094001;-0.00066 -1.15922103401065e-09 -5298.04671731616 -1918.07482852342;-0.0006 -1.15990077992839e-09 -5253.3088472621 -2037.41352512251;-0.00054 -1.15998709917463e-09 -5205.8832873318 -2155.70984331509;-0.00048 -1.15947994758682e-09 -5155.79430131804 -2272.90326051888;-0.00042 -1.15837958463311e-09 -5103.06751567159 -2388.93381841617;-0.00036 -1.1566865732795e-09 -5047.72990639029 -2503.74215362953;-0.0003 -1.15440177970189e-09 -4989.80978521755 -2617.26952809327;-0.00024 -1.1515263728429e-09 -4929.3367851576 -2729.45785910485;-0.00018 -1.1480618238138e-09 -4866.3418453147 -2840.24974904113;-0.00012 -1.14400990514189e-09 -4800.85719506408 -2949.58851472402;-6e-05 -1.13937268986364e-09 -4732.91633756282 -3057.41821642064]  x4=[-0.00138 1.08340244121566e-09 -4645.9302356518 -6447.87208957731;-0.00132 1.11152986981396e-09 -4498.90652702436 -6551.30302319254;-0.00126 1.13908861919215e-09 -4349.58109468746 -6651.38218912695;-0.0012 1.16606458978483e-09 -4198.0303362915 -6748.05838502999;-0.00114 1.19244398018698e-09 -4044.33178800481 -6841.28214957347;-0.00108 1.21821329421503e-09 -3888.56408484472 -6931.00578775686;-0.00102 1.24335934781176e-09 -3730.80692044642 -7017.18339530898;-0.00096 1.26786927579152e-09 -3571.14100629023 -7099.77088217341;-0.0009 1.29173053842225e-09 -3409.64803040813 -7178.72599506585;-0.00084 1.31493092784109e-09 -3246.41061559062 -7254.0083390916;-0.00078 1.33745857430012e-09 -3081.5122771154 -7325.57939841241;-0.00072 1.35930195223914e-09 -2915.03738001941 -7393.40255595185;-0.00066 1.38044988618238e-09 -2747.0710959361 -7457.44311212929;-0.0006 1.40089155645607e-09 -2577.69935952007 -7517.66830261286;-0.00054 1.42061650472398e-09 -2407.00882448131 -7574.04731508228;-0.00048 1.43961463933809e-09 -2235.08681925153 -7626.551304993;-0.00042 1.4578762405017e-09 -2062.02130230537 -7675.15341033361;-0.00036 1.47539196524222e-09 -1887.90081715917 -7719.82876536898;-0.0003 1.49215285219121e-09 -1712.81444707052 -7760.55451336194;-0.00024 1.5081503261692e-09 -1536.85176946158 -7797.30981826731;-0.00018 1.52337620257291e-09 -1360.10281008962 -7830.07587539193;-0.00012 1.53782269156263e-09 -1182.65799698822 -7858.83592101554;-6e-05 1.55148240204764e-09 -1004.60811420254 -7883.57524096736]  x5=0.00132336726677004  V1=[5.094e-16 1.649e-05 1.649e-05;377 377 377;1.389 -1.935 2.777]  V2=[3.793e-13 0.4417 0.4417;377 377 377;-0.7025 -1.967 2.745]  I1=[9.917e-16 0.005412 0.005412;377 377 377;-2.043 2.781 1.21]  I2=[8.773e-16 0.005353 0.005353;377 377 377;0.5828 -0.6661 -2.237]  nHarmo=1  Measurements=None  Decoupling=off  VsMag0=0  VrMag0=0  VsAngle0=0  VrAngle0=0  IsMag0=0  IrMag0=0  IsAngle0=0  IrAngle0=0
      settings: LibrarySourceBlock=sps_lib/Power Grid Elements/Distributed Parameters Line
  MPP7 4700 MVA 17KV : spsSynchronousMachinepuStandardLib/Synchronous Machine pu Standard  PresetModel=No  MechanicalLoad=Mechanical power Pm  ShowDetailedParameters=on  RotorType=Salient-pole  Units=per unit standard parameters  MeasurementBus=off  NominalParameters=[2700e6 17000 60]  Reactances1=[ 1.81, 0.3, 0.23, 1.76, 0.65, 0.25, 0.15 ]  Reactances2=[ 1.305, 0.296, 0.252, 0.474, 0.243, 0.18 ]  dAxisTimeConstants=Short-circuit  qAxisTimeConstants=Open-circuit  TimeConstants1="[ 4.4849  0.0681  0.1  ]"  TimeConstants2=[ 8.0, 0.03, 1.0, 0.07 ]  TimeConstants3="[  4.49  0.0681  0.0513  ]"  TimeConstants4=[ 8.0, 0.03, 0.3371, 0.0295 ]  TimeConstants5=[ 1.01, 0.053, 0.1 ]  TimeConstants6=[ 1.3201, 0.023, 1.0, 0.07 ]  TimeConstants7=[0.012 0.003 0.003]  TimeConstants8=[ 1.3201, 0.0231, 0.3371, 0.0295 ]  StatorResistance=2.8544e-3  Mechanical=[3.5 0 32]  PolePairs=20  InitialConditions=[0 -81.9543 0.907703 0.907703 0.907703 -8.76021 -128.76 111.24 1.25655]  SetSaturation=off  Saturation=[0.6404,0.7127,0.8441,0.9214,0.9956,1.082,1.19,1.316,1.457;0.7,0.7698,0.8872,0.9466,0.9969,1.046,1.1,1.151,1.201]  LoadFlowParameters=[1,0,0,0,0]  TsPowergui=0  TsBlock=-1  IterativeModel=Trapezoidal non iterative  IterativeDiscreteModel=Trapezoidal non iterative  BusType=PV  Pref=3845e6  Qref=0  Qmin=-inf  Qmax=inf  PLF=0  QLF=0
  MTL Load : Subsystem
  NAN 1 : spsThreePhaseVIMeasurementLib/Three-Phase V-I Measurement  VoltageMeasurement=phase-to-ground  SetLabelV=on  LabelV=Vabc_NAN1  Vpu=off  VpuLL=off  CurrentMeasurement=no  SetLabelI=off  LabelI=Iabc  Ipu=off  Pbase=100e6  Vbase=500e3  OutputType=Complex  PhasorSimulation=off  PSBequivalent=0
  NAN-SAT 109 km : spsDistributedParametersLineLib/Distributed Parameters Line  Phases=3  Length=109  Frequency=60  Resistance=[0.01273 0.3864]/6  Inductance="[0.9337e-3  4.1264e-3]/6"  Capacitance=[12.74e-9 7.751e-9]*6  x1=[-0.00066 3.9051050709363e-08 0 0;-0.0006 4.00910071741062e-08 0 0;-0.00054 4.11104523387824e-08 0 0;-0.00048 4.21088646364083e-08 0 0;-0.00042 4.30857332608039e-08 -59331.3571758165 -190971.332944293;-0.00036 4.40405584279304e-08 -54996.8795763366 -192264.439145427;-0.0003 4.49728516315892e-08 -50634.2645570399 -193459.179306856;-0.00024 4.58821358933506e-08 -46245.7441123822 -194554.942177436;-0.00018 4.67679460065845e-08 -41833.5634905135 -195551.167144637;-0.00012 4.76298287744692e-08 -37399.9800445677 -196447.344521356;-6e-05 4.84673432418548e-08 -32947.2620777589 -197243.015806689]  x2=[-0.00066 8.6277623494704e-09 0 0;-0.0006 8.38512951862173e-09 0 0;-0.00054 8.13820670057196e-09 0 0;-0.00048 7.8871202255974e-09 0 0;-0.00042 7.63199855417821e-09 -119627.728475328 -210779.530785662;-0.00036 7.37297221127558e-09 -114829.810775075 -213431.327940766;-0.0003 7.11017371955279e-09 -109973.144021819 -215973.929684739;-0.00024 6.84373753157418e-09 -105060.212976012 -218406.035175546;-0.00018 6.57379996101669e-09 -100093.531183956 -220726.400103077;-0.00012 6.30049911292928e-09 -95075.6396918308 -222933.837325761;-6e-05 6.02397481307586e-09 -90009.1057456434 -225027.217477925]  x3=[-0.00066 1.88362985523887e-09 0 0;-0.0006 1.85944391651348e-09 0 0;-0.00054 1.83430665192183e-09 0 0;-0.00048 1.80823092215297e-09 0 0;-0.00042 1.78123006803207e-09 -5045.05844095481 5189.76090253494;-0.00036 1.75331790369502e-09 -5161.14704709689 5074.32632806901;-0.0003 1.72450870952084e-09 -5274.59511504265 4956.29563449087;-0.00024 1.69481722482562e-09 -5385.34460266424 4835.72920848432;-0.00018 1.66425864032156e-09 -5493.33884847738 4712.6887340607;-0.00012 1.63284859034514e-09 -5598.52260063041 4587.23716100026;-6e-05 1.60060314485833e-09 -5700.84204517215 4459.43867264585]  x4=[-0.00066 -1.54492520971202e-09 0 0;-0.0006 -1.51348214435974e-09 0 0;-0.00054 -1.48126475357647e-09 0 0;-0.00048 -1.44828952037465e-09 0 0;-0.00042 -1.41457331549289e-09 463.588669967568 -13778.8122021793;-0.00036 -1.38013338876462e-09 775.112558842218 -13764.8033824906;-0.0003 -1.34498736029272e-09 1086.23988580933 -13743.7522350471;-0.00024 -1.30915321143479e-09 1396.81147237946 -13715.6695300048;-0.00018 -1.27264927560352e-09 1706.66842439021 -13680.5696349945;-0.00012 -1.23549422888699e-09 2015.65221329944 -13638.4705077711;-6e-05 -1.19770708049365e-09 2323.60475729137 -13589.3936870259]  x5=0.000616440308025359  V1=[4.327e-18 2.694e-07 2.694e-07;377 377 377;-0.06841 1.312 -0.2585]  V2=[4.095e-15 0.006804 0.006804;377 377 377;-0.7508 1.28 -0.2912]  I1=[2.296e-17 0.0001774 0.0001774;377 377 377;-2.081 -0.2552 -1.826]  I2=[2.168e-17 0.0001764 0.0001764;377 377 377;0.8233 2.744 1.174]  nHarmo=1  Measurements=None  Decoupling=off  VsMag0=0  VrMag0=0  VsAngle0=0  VrAngle0=0  IsMag0=0  IrMag0=0  IsAngle0=0  IrAngle0=0
      settings: LibrarySourceBlock=sps_lib/Power Grid Elements/Distributed Parameters Line
  North Network : Subsystem
  ORE-NAN 117 km3 : spsDistributedParametersLineLib/Distributed Parameters Line  Phases=3  Length=117  Frequency=60  Resistance=[0.01273 0.3864]/6  Inductance="[0.9337e-3  4.1264e-3]/6"  Capacitance=[12.74e-9 7.751e-9]*6  x1=[-0.00072 -3.28001082988995e-09 0 0;-0.00066 -3.61104883623502e-09 0 0;-0.0006 -3.94023936327096e-09 0 0;-0.00054 -4.2674139910414e-09 0 0;-0.00048 -4.59240533096127e-09 0 0;-0.00042 -4.91504711145593e-09 -79334.9684638627 -197415.798616379;-0.00036 -5.23517426302875e-09 -74849.6146942539 -199159.689133432;-0.0003 -5.5526230027137e-09 -70325.9664787057 -200801.685873476;-0.00024 -5.86723091786978e-09 -65766.3381992325 -202340.948760638;-0.00018 -6.17883704927432e-09 -61173.0626459144 -203776.690279584;-0.00012 -6.48728197347267e-09 -56548.4898233984 -205108.175878422;-6e-05 -6.7924078843422e-09 -51894.9857485927 -206334.724344517]  x2=[-0.00072 8.86598105767836e-09 0 0;-0.00066 8.6277623494704e-09 0 0;-0.0006 8.38512951862173e-09 0 0;-0.00054 8.13820670057196e-09 0 0;-0.00048 7.8871202255974e-09 0 0;-0.00042 7.63199855417821e-09 -119627.728475328 -210779.530785662;-0.00036 7.37297221127558e-09 -114829.810775075 -213431.327940766;-0.0003 7.11017371955279e-09 -109973.144021819 -215973.929684739;-0.00024 6.84373753157418e-09 -105060.212976012 -218406.035175546;-0.00018 6.57379996101669e-09 -100093.531183956 -220726.400103077;-0.00012 6.30049911292928e-09 -95075.6396918308 -222933.837325761;-6e-05 6.02397481307586e-09 -90009.1057456434 -225027.217477925]  x3=[-0.00072 -4.61025874789674e-11 0 0;-0.00066 -3.97360044498687e-11 0 0;-0.0006 -3.33490917466565e-11 0 0;-0.00054 -2.69451170318864e-11 0 0;-0.00048 -2.05273566973542e-11 0 0;-0.00042 -1.40990941878338e-11 -4241.41632083877 1575.36871122334;-0.00036 -7.66361832120551e-12 -4275.96191997411 1479.0349393088;-0.0003 -1.22422160583673e-12 -4308.3198579805 1381.94446578988;-0.00024 5.21580144392661e-12 -4338.47357993895 1284.14696394686;-0.00018 1.16531559932943e-11 -4366.40765864813 1185.69246878879;-0.00012 1.80845485727303e-11 -4392.10780251721 1086.6313514546;-6e-05 2.45066887629524e-11 -4415.56086287769 987.01429344237]  x4=[-0.00072 1.19771949205318e-10 0 0;-0.00066 1.08966119319193e-10 0 0;-0.0006 9.81045403529625e-11 0 0;-0.00054 8.71927692911235e-11 0 0;-0.00048 7.62363887973782e-11 0 0;-0.00042 6.52410043584375e-11 -837.617553665554 -10249.8207998506;-0.00036 5.4212241416152e-11 -605.577802394573 -10266.1446186628;-0.0003 4.31557424894308e-11 -373.228226330095 -10277.2160881916;-0.00024 3.20771642874257e-11 -140.687699808562 -10283.0295440685;-0.00018 2.09821748154533e-11 91.9248051398026 -10283.5820120221;-0.00012 9.87645047513924e-12 324.490279659283 -10278.8732093997;-6e-05 -1.23432683973369e-12 556.889738955798 -10268.9055453116]  x5=0.000661683633385019  V1=[2.771e-15 0.004375 0.004375;377 377 377;-0.7831 1.268 -0.3032]  V2=[4.095e-15 0.006804 0.006804;377 377 377;-0.7678 1.269 -0.3016]  I1=[9.029e-18 6.296e-05 6.296e-05;377 377 377;-1.689 -0.005215 -1.576]  I2=[6.955e-18 6.141e-05 6.141e-05;377 377 377;0.2743 2.461 0.89]  nHarmo=1  Measurements=None  Decoupling=off  VsMag0=0  VrMag0=0  VsAngle0=0  VrAngle0=0  IsMag0=0  IrMag0=0  IsAngle0=0  IrAngle0=0
      settings: LibrarySourceBlock=sps_lib/Power Grid Elements/Distributed Parameters Line
  OSI 1 : spsThreePhaseVIMeasurementLib/Three-Phase V-I Measurement  VoltageMeasurement=no  SetLabelV=on  LabelV=Vabc  Vpu=off  VpuLL=off  CurrentMeasurement=no  SetLabelI=off  LabelI=Iabc  Ipu=off  Pbase=100e6  Vbase=500e3  OutputType=Complex  PhasorSimulation=off  PSBequivalent=0
  OSI-MPO 187 km : spsDistributedParametersLineLib/Distributed Parameters Line  Phases=3  Length=187  Frequency=60  Resistance=[0.01273 0.3864]/6  Inductance="[0.9337e-3  4.1264e-3]/6"  Capacitance=[12.74e-9 7.751e-9]*6  x1=[-0.00108 8.34832245833401e-09 0 0;-0.00102 1.05781884249661e-08 0 0;-0.00096 1.28026423949375e-08 0 0;-0.0009 1.50205462964941e-08 0 0;-0.00084 1.72307654090175e-08 0 0;-0.00078 1.94321689435698e-08 0 0;-0.00072 2.16236306214254e-08 0 0;-0.00066 2.38040292502962e-08 -160574.30309592 -252154.438296983;-0.0006 2.59722492979548e-08 -154830.108476143 -255721.76777496;-0.00054 2.81271814629605e-08 -149006.699911937 -259158.265271348;-0.00048 3.02677232421992e-08 -143107.05676673 -262462.172610529;-0.00042 3.2392779494944e-08 -137134.197406966 -265631.799452459;-0.00036 3.45012630031494e-08 -131091.177657861 -268665.524157478;-0.0003 3.65920950276924e-08 -124981.089239979 -271561.79461597;-0.00024 3.8664205860275e-08 -118807.058187457 -274319.129042452;-0.00018 4.07165353707071e-08 -112572.243248664 -276936.11673368;-0.00012 4.27480335492885e-08 -106279.834270129 -279411.418790397;-6e-05 4.47576610440133e-08 -99933.0505645563 -281743.768802331]  x2=[-0.00108 -3.45195330620732e-09 0 0;-0.00102 -1.26821480186422e-09 0 0;-0.00096 9.16172544605432e-10 0 0;-0.0009 3.10009116027235e-09 0 0;-0.00084 5.28242371201856e-09 0 0;-0.00078 7.46205367818575e-09 0 0;-0.00072 9.63786591980827e-09 0 0;-0.00066 1.18087472511389e-08 -164760.640389433 -246825.53367241;-0.0006 1.39735870091754e-08 -159135.901182384 -250488.909407147;-0.00054 1.61312776218957e-08 -153429.745107798 -254024.130387328;-0.00048 1.82807151749129e-08 -147645.091540558 -257429.387928577;-0.00042 2.04207999762579e-08 -141784.900016319 -260702.939838213;-0.00036 2.2550437119002e-08 -135852.168717347 -263843.111306591;-0.0003 2.46685370414318e-08 -129849.932938601 -266848.295763965;-0.00024 2.67740160844891e-08 -123781.263534812 -269716.955702437;-0.00018 2.88657970461907e-08 -117649.265349384 -272447.623462575;-0.00012 3.09428097327448e-08 -111457.075625894 -275038.901984296;-6e-05 3.30039915060823e-08 -105207.862403025 -277489.465521627]  x3=[-0.00108 -1.02748071515385e-10 0 0;-0.00102 -9.07084902045292e-11 0 0;-0.00096 -7.86225007539851e-11 0 0;-0.0009 -6.64962865792783e-11 0 0;-0.00084 -5.43360516756476e-11 0 0;-0.00078 -4.21480174439647e-11 0 0;-0.00072 -2.99384195077518e-11 0 0;-0.00066 -1.77135045229203e-11 -3741.02213218041 -4718.13443168593;-0.0006 -5.47952698186686e-12 -3633.35247695178 -4801.54096983384;-0.00054 6.75725398644047e-12 -3523.8239314593 -4882.49095089931;-0.00048 1.89905778187486e-11 -3412.49253253071 -4960.94295937624;-0.00042 3.12141857205392e-11 -3299.41523936687 -5036.85685776747;-0.00036 4.34218238681433e-11 -3184.64990440038 -5110.19380711985;-0.0003 5.56072466083134e-11 -3068.25524369723 -5180.91628689498;-0.00024 6.77642196536149e-11 -2950.29080691658 -5248.98811416541;-0.00018 7.98865232720028e-11 -2830.81694684399 -5314.37446212648;-0.00012 9.19679554689515e-11 -2709.89478851392 -5377.04187791438;-6e-05 1.0400233516051e-10 -2587.58619793695 -5436.95829972123]  x4=[-0.00108 -1.67233330749075e-10 0 0;-0.00102 -1.45343744839331e-10 0 0;-0.00096 -1.23379798384084e-10 0 0;-0.0009 -1.01352728544188e-10 0 0;-0.00084 -7.92738047755845e-11 0 0;-0.00078 -5.71543230636467e-11 0 0;-0.00072 -3.50056001439391e-11 0 0;-0.00066 -1.28389677123688e-11 -4767.01630034413 -5390.75196404232;-0.0006 9.33423337232008e-12 -4643.87094424703 -5497.19194850936;-0.00054 3.15026588907389e-11 -4518.349697966 -5600.81946799912;-0.00048 5.36549670667669e-11 -4390.51678048998 -5701.5815047578;-0.00042 7.57798243702138e-11 -4260.43759350164 -5799.42650706554;-0.00036 9.78659113152628e-11 -4128.17868791663 -5894.30441561118;-0.0003 1.19901928251729e-10 -3993.80772983491 -5986.16668910357;-0.00024 1.41876601146168e-10 -3857.39346592152 -6074.96632910618;-0.00018 1.63778687349883e-10 -3719.00568823453 -6160.65790408234;-0.00012 1.85596981350868e-10 -3578.71519851812 -6243.1975726389;-6e-05 2.07320320506755e-10 -3436.59377197909 -6322.54310595628]  x5=0.00105756273028204  V1=[3.05e-13 0.3186 0.3186;377 377 377;-0.6471 -1.909 2.804]  V2=[3.793e-13 0.4417 0.4417;377 377 377;-0.6023 -1.906 2.806]  I1=[5.824e-16 0.002377 0.002377;377 377 377;-1.191 -2.924 1.788]  I2=[4.03e-16 0.002279 0.002279;377 377 377;-0.283 -1.078 -2.649]  nHarmo=1  Measurements=None  Decoupling=off  VsMag0=0  VrMag0=0  VsAngle0=0  VrAngle0=0  IsMag0=0  IrMag0=0  IsAngle0=0  IrAngle0=0
      settings: LibrarySourceBlock=sps_lib/Power Grid Elements/Distributed Parameters Line
  PSS : Constant
  PSS_Equation : Subsystem
  Regulators 10 : Subsystem
  South Network : Subsystem
  Stair Generator : eeStairGenerator/Stair Generator  LabelModeActiveChoice=Discrete  TimeInput=[0.1 0.15 0.2]  AmplitudeInput=[0 1 0]  SampleTime=-1  RepeatPattern=off  OutDataTypeStr=double
      settings: LibrarySourceBlock=ee_sl_lib/General Control/Stair Generator
  Three-Phase Fault : spsThreePhaseFaultLib/Three-Phase Fault  InitialStates=0  FaultA=on  FaultB=on  FaultC=on  GroundFault=on  SwitchTimes="[0.2  0.4]"  External=on  SwitchStatus=NaN  FaultResistance=0.001  GroundResistance=0.01  SnubberResistance=1e6  SnubberCapacitance=inf  Measurements=None
  powergui : sps_lib/powergui  Priority=1  SimulationMode=Discrete  SampleTime=6e-5  frequency=60  Iterations=50  frequencyindice=60  Pbase=100e6  ErrMax=1e-4  UnitsV=kV  UnitsW=MW  buscounter=0  FunctionMessages=off  echomessages=off  EnableUseOfTLC=off  CurrentSourceSwitches=off  DisableSnubberDevices=off  DisableRonSwitches=off  DisableVfSwitches=off  DisplayEquations=off  AutomaticDiscreteSolvers=off  SolverType=Tustin/Backward Euler (TBE)  Interpol=off  ExternalGateDelay=off  methode=off  Ts=100  x0status=blocks  SPID=on  SwTol=0  HookPort=off  NonlinearTolerance=1e-4  nMaxIteration=100  ContinueOnMaxIteration=off  RestoreLinks=warning  ResistiveCurrentMeasurement=off  Frange=[0:2:500]  Ylog=off  Xlog=on  ShowGrid=off  save=off  variable=ZData  structure=0  ZoomFFT=off  StartTime=0.0  cycles=1  DisplayStyle=1  fundamental=60  FreqAxis=off  MaxFrequency=1000  frequencyindicesteady=1  RmsSteady=1  display=off
  wires:
  PSS/1 -> PSS_Equation/1(In1)
  Regulators 10/1(Pm) -> MPP7 4700 MVA 17KV/1
  MPP7 4700 MVA 17KV/1 -> Regulators 10/1(m)
  Regulators 10/2(Vf) -> MPP7 4700 MVA 17KV/2
  Stair Generator/1 -> Three-Phase Fault/1
  connections:
  South Network/LConn3 -- CON-OSI 144 km/RConn3
  South Network/LConn2 -- CON-OSI 144 km/RConn2
  South Network/LConn1 -- CON-OSI 144 km/RConn1
  OSI 1/LConn1 -- CON-OSI 144 km/LConn1
  CON-OSI 144 km/LConn2 -- OSI 1/LConn2
  CON-OSI 144 km/LConn3 -- OSI 1/LConn3
  Cs OSIS/LConn1 -- OSI 1/RConn1
  Cs OSIS/LConn2 -- OSI 1/RConn2
  Cs OSIS/LConn3 -- OSI 1/RConn3
  150 MW/LConn1 -- MPP7 4700 MVA 17KV/RConn1 -- "4700 MVA 17KV :650KV Transformer "/LConn1 -- Load Flow Bus1/LConn1
  150 MW/LConn2 -- MPP7 4700 MVA 17KV/RConn2 -- "4700 MVA 17KV :650KV Transformer "/LConn2
  "4700 MVA 17KV :650KV Transformer "/LConn3 -- MPP7 4700 MVA 17KV/RConn3 -- 150 MW/LConn3
  North Network/RConn1 -- ATL-MPO 350 km/RConn1
  Cs OSIS/RConn1 -- Load Flow Bus3/LConn1 -- OSI-MPO 187 km/LConn1
  Cs OSIS/RConn2 -- OSI-MPO 187 km/LConn2
  Cs OSIS/RConn3 -- OSI-MPO 187 km/LConn3
  MPP10-MPO 234 km/LConn1 -- 330 MVar/LConn1 -- "4700 MVA 17KV :650KV Transformer "/RConn1
  MPP10-MPO 234 km/LConn2 -- 330 MVar/LConn2 -- "4700 MVA 17KV :650KV Transformer "/RConn2
  MPP10-MPO 234 km/LConn3 -- "4700 MVA 17KV :650KV Transformer "/RConn3 -- 330 MVar/LConn3
  MPP10-MPO 234 km/RConn1 -- " Wind Generation + Load"/LConn1 -- OSI-MPO 187 km/RConn1 -- 400 kV Solar Farm/LConn1 -- Cs MPOD/RConn1 -- Load Flow Bus2/LConn1
  MPP10-MPO 234 km/RConn2 -- 400 kV Solar Farm/LConn2 -- " Wind Generation + Load"/LConn2 -- OSI-MPO 187 km/RConn2 -- Cs MPOD/RConn2
  MPP10-MPO 234 km/RConn3 -- " Wind Generation + Load"/LConn3 -- OSI-MPO 187 km/RConn3 -- 400 kV Solar Farm/LConn3 -- Cs MPOD/RConn3
  MPO 3/RConn1 -- ATL-MPO 350 km/LConn1 -- Cs MPOD/LConn1
  MPO 3/RConn2 -- ATL-MPO 350 km/LConn2 -- Cs MPOD/LConn2
  MPO 3/RConn3 -- ATL-MPO 350 km/LConn3 -- Cs MPOD/LConn3
  NAN 1/LConn2 -- Home Network Load （with circuit breaker)/LConn2 -- MTL Load/LConn2 -- Three-Phase Fault/LConn2 -- NAN-SAT 109 km/RConn2 -- MPO-NAN 277 km/RConn2
  MTL Load/LConn1 -- Home Network Load （with circuit breaker)/LConn1 -- Three-Phase Fault/LConn1 -- Load Flow Bus4/LConn1 -- NAN-SAT 109 km/RConn1 -- MPO-NAN 277 km/RConn1 -- NAN 1/LConn1 -- Load Flow Bus5/LConn1
  ATL-MPO 350 km/RConn2 -- North Network/RConn2
  North Network/RConn3 -- ATL-MPO 350 km/RConn3
  North Network/LConn1 -- ORE-NAN 117 km3/LConn1
  North Network/LConn2 -- ORE-NAN 117 km3/LConn2
  North Network/LConn3 -- ORE-NAN 117 km3/LConn3
  NAN 1/RConn3 -- ORE-NAN 117 km3/RConn3
  ORE-NAN 117 km3/RConn2 -- NAN 1/RConn2
  ORE-NAN 117 km3/RConn1 -- NAN 1/RConn1
  South Network/LConn4 -- NAN-SAT 109 km/LConn1
  South Network/LConn5 -- NAN-SAT 109 km/LConn2
  South Network/LConn6 -- NAN-SAT 109 km/LConn3
  MPO-NAN 277 km/LConn3 -- 660 MVar/LConn3 -- MPO 3/LConn3
  MPO 3/LConn2 -- 660 MVar/LConn2 -- MPO-NAN 277 km/LConn2
  MPO-NAN 277 km/LConn1 -- 660 MVar/LConn1 -- MPO 3/LConn1
  MPO-NAN 277 km/RConn3 -- NAN-SAT 109 km/RConn3 -- Home Network Load （with circuit breaker)/LConn3 -- MTL Load/LConn3 -- Three-Phase Fault/LConn3 -- NAN 1/LConn3
